simulink model "Caracteriza_Motor"  (R2023a)
settings: Solver=VariableStepAuto  StartTime=0.0  StopTime=2  RelTol=1e-3
values from neighbouring files (symbols this model uses):
  a = zeta*2*sqrt(kp*k)    [teste.m]
  k = Wn^2/kp    [teste.m]
  kp = 4.5    [teste.m]
settings Model: Creator=hiago.sodre  LastModifiedBy=hiago.sodre

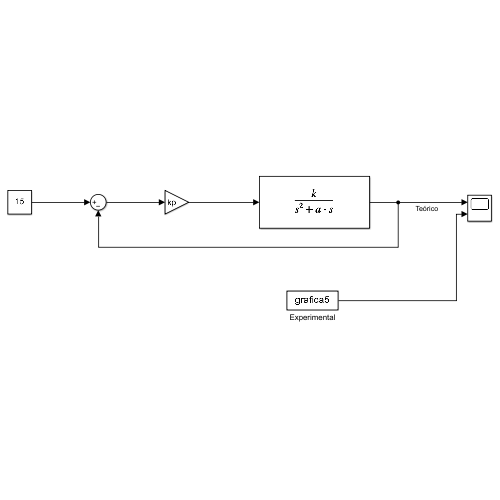
[thumbnail: Simulink's stored preview of the top-level diagram]
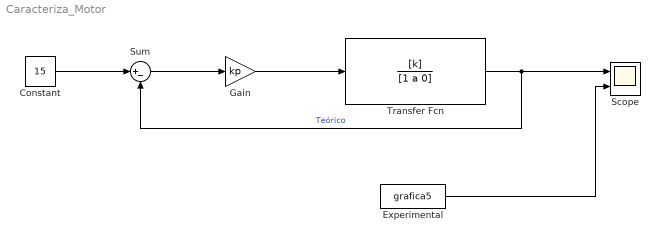
== system Caracteriza_Motor ==
  Constant : Constant  Value=15
  Experimental : FromWorkspace  VariableName=grafica5
  Gain : Gain  Gain=kp
  Scope : Scope  NumInputPorts=2
  Sum : Sum  Inputs=|+-
  Transfer Fcn : TransferFcn  Numerator=[k]  Denominator=[1 a 0]  ParameterTunability=Unconstrained
  wires:
  Experimental/1 -> Scope/2
  Gain/1 -> Transfer Fcn/1
  Sum/1 -> Gain/1
  Transfer Fcn/1 -> Scope/1, Sum/2  "Teórico"
  Constant/1 -> Sum/1
